simulink model "HalfCar"  (R2024b)
settings: Solver=VariableStepAuto  StartTime=0.0  StopTime=20  RelTol=1e-3
libraries: simulink x12
settings Model: Creator=Seb  LastModifiedBy=sebam

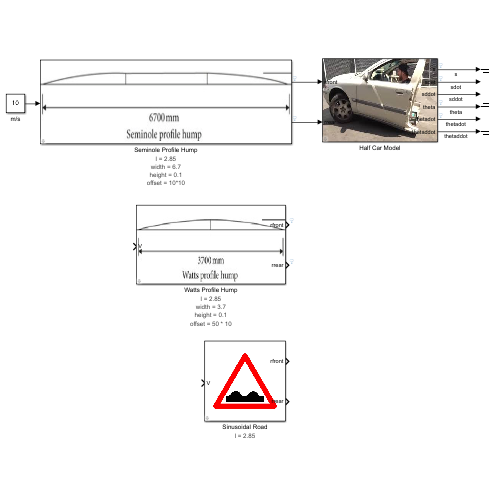
[thumbnail: Simulink's stored preview of the top-level diagram]
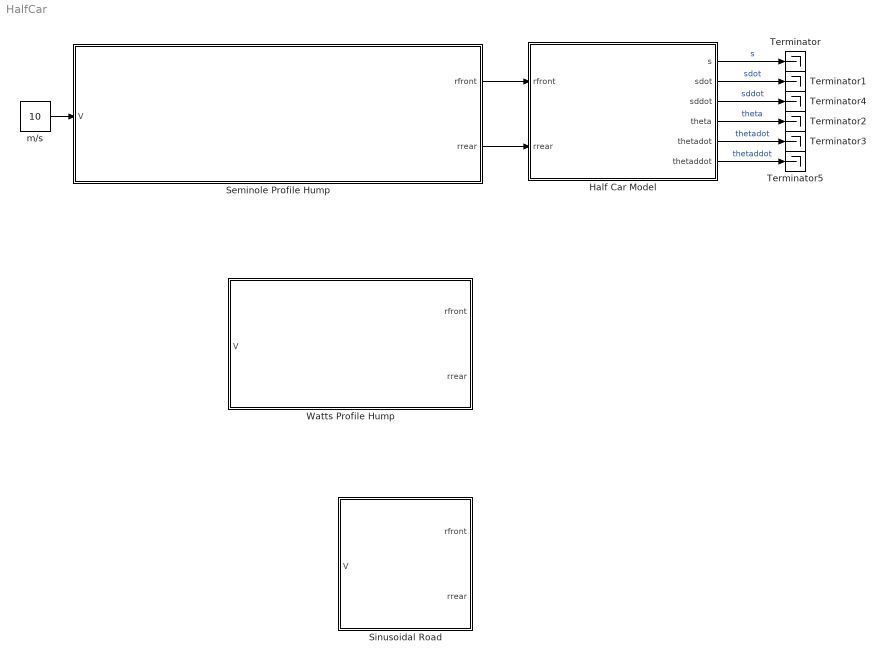
== system HalfCar ==
  Half Car Model : Subsystem
      mask Display: image('car.jpg');
  Seminole Profile Hump : Subsystem  mask{l=2.85, width=6.7, height=0.1, offset=10*10}
      mask prompts: l "Wheelbase (l)"; width "Hump Width (width)"; height "Hump Height (height)"; offset "Hump Offset (offset)"
      settings: AttributesFormatString=|
      | l = %<l>
      | width = %<width>
      | height = %<height>
      | offset = %<offset>
      mask Display: image('seminole.png');
  Sinusoidal Road : Subsystem  mask{l=2.85}
      mask prompts: l "Wheelbase (l)"
      settings: AttributesFormatString=l = %<l>
      mask Display: image('road.jpg');
  Terminator{,1..5} (6 alike) : Terminator
  Watts Profile Hump : Subsystem  mask{l=2.85, width=3.7, height=0.1, offset=50 * 10}
      mask prompts: l "Wheelbase (l)"; width "Hump Width (width)"; height "Hump Height (height)"; offset "Hump Offset (offset)"
      settings: AttributesFormatString=|
      | l = %<l>
      | width = %<width>
      | height = %<height>
      | offset = %<offset>
      mask Display: image('watt.png');
  m/s : Constant  Value=10
  wires:
  Half Car Model/1(s) -> Terminator/1  "s"
  Half Car Model/2(sdot) -> Terminator1/1  "sdot"
  Half Car Model/4(theta) -> Terminator2/1  "theta"
  Half Car Model/5(thetadot) -> Terminator3/1  "thetadot"
  m/s/1 -> Seminole Profile Hump/1(V)
  Seminole Profile Hump/1(rfront) -> Half Car Model/1(rfront)
  Seminole Profile Hump/2(rrear) -> Half Car Model/2(rrear)
  Half Car Model/3(sddot) -> Terminator4/1  "sddot"
  Half Car Model/6(thetaddot) -> Terminator5/1  "thetaddot"

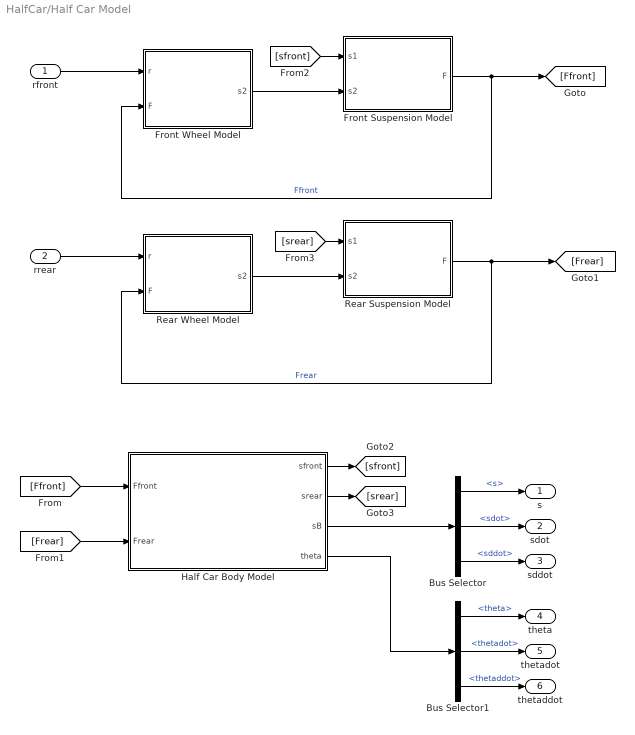
== system HalfCar/Half Car Model ==
  rfront : Inport
  rrear : Inport  Port=2
  Bus Selector : BusSelector  OutputSignals=s,sdot,sddot
  Bus Selector1 : BusSelector  OutputSignals=theta,thetadot,thetaddot
  Front Suspension Model : Subsystem  mask{ks=2e4, k2=20*2e4, x0=0.2, ce=1200, cc=600}
      mask prompts: ks "Spring Stiffness (ks)"; k2 "Spring Hardening Stiffness (k2)"; x0 "Spring Hardening Location (x0)"; ce "Damping Rate Extension (cse)"; cc "Damping Rate Compression (csc)"
      settings: AttributesFormatString=|
      | ks = %<ks>
      | k2 = %<k2>
      | x0 = %<x0>
      | ce = %<ce>
      | cc = %<cc>
      mask Display: fprintf("Suspension\nModel")
  Front Wheel Model : Subsystem  mask{m2=20, g=9.81, kT=14e4}
      mask prompts: m2 "Mass (m2)"; g "Gravity (g)"; kT "Wheel Stiffness (kT)"
      settings: AttributesFormatString=|
      | g = %<g>
      | kT = %<kT>
      | m2 = %<m2>
      mask Display: fprintf("Wheel\nModel")
  Half Car Body Model : Subsystem  mask{mB=700, IB=650, g=9.81, a=1.35, b=1.5}
      mask prompts: mB "Mass (mB)"; IB "Moment of Inertia (IB)"; g "Gravity (g)"; a "Length A (a)"; b "Length B (b)"
      settings: AttributesFormatString=|
      | mB = %<mB>
      | IB = %<IB>
      | g = %<g>
      | a = %<a>
      | b = %<b>
      mask Display: fprintf("Half Car\nBody Model")
  Rear Suspension Model : Subsystem  mask{ks=2e4, k2=20*2e4, x0=0.2, ce=1200, cc=600}
      mask prompts: ks "Spring Stiffness (ks)"; k2 "Spring Hardening Stiffness (k2)"; x0 "Spring Hardening Location (x0)"; ce "Damping Rate Extension (cse)"; cc "Damping Rate Compression (csc)"
      settings: AttributesFormatString=|
      | ks = %<ks>
      | k2 = %<k2>
      | x0 = %<x0>
      | ce = %<ce>
      | cc = %<cc>
      mask Display: fprintf("Suspension\nModel")
  Rear Wheel Model : Subsystem  mask{m2=20, g=9.81, kT=14e4}
      mask prompts: m2 "Mass (m2)"; g "Gravity (g)"; kT "Wheel Stiffness (kT)"
      settings: AttributesFormatString=|
      | g = %<g>
      | kT = %<kT>
      | m2 = %<m2>
      mask Display: fprintf("Wheel\nModel")
  s : Outport
  sdot : Outport  Port=2
  sddot : Outport  Port=3
  theta : Outport  Port=4
  thetadot : Outport  Port=5
  thetaddot : Outport  Port=6
  wires:
  Front Wheel Model/1(s2) -> Front Suspension Model/2(s2)
  Half Car Body Model/3(sB) -> Bus Selector/1
  Front Suspension Model/1(F) -> [Ffront], Front Wheel Model/2(F)  "Ffront"
  Bus Selector/2 -> sdot/1  "<sdot>"
  Half Car Body Model/4(theta) -> Bus Selector1/1
  Bus Selector1/1 -> theta/1  "<theta>"
  rfront/1 -> Front Wheel Model/1(r)
  Bus Selector1/2 -> thetadot/1  "<thetadot>"
  rrear/1 -> Rear Wheel Model/1(r)
  Bus Selector/1 -> s/1  "<s>"
  Rear Suspension Model/1(F) -> [Frear], Rear Wheel Model/2(F)  "Frear"
  Rear Wheel Model/1(s2) -> Rear Suspension Model/2(s2)
  [Ffront] -> Half Car Body Model/1(Ffront)
  [Frear] -> Half Car Body Model/2(Frear)
  Half Car Body Model/1(sfront) -> [sfront]
  Half Car Body Model/2(srear) -> [srear]
  [sfront] -> Front Suspension Model/1(s1)
  [srear] -> Rear Suspension Model/1(s1)
  Bus Selector/3 -> sddot/1  "<sddot>"
  Bus Selector1/3 -> thetaddot/1  "<thetaddot>"

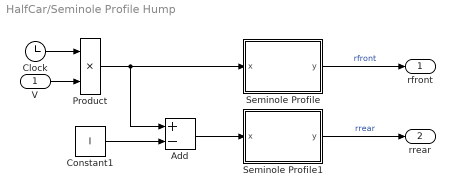
== system HalfCar/Seminole Profile Hump ==
  V : Inport
  Add : Sum  Inputs=+-
  Clock : Clock
  Constant1 : Constant  Value=l
  Product : Product
  Seminole Profile : Subsystem
  Seminole Profile1 : Subsystem
  rfront : Outport
  rrear : Outport  Port=2
  wires:
  V/1 -> Product/2
  Seminole Profile1/1(y) -> rrear/1  "rrear"
  Constant1/1 -> Add/2
  Product/1 -> Seminole Profile/1(x), Add/1
  Add/1 -> Seminole Profile1/1(x)
  Seminole Profile/1(y) -> rfront/1  "rfront"
  Clock/1 -> Product/1

== system HalfCar/Sinusoidal Road ==
  V : Inport
  Add : Sum  Inputs=+-
  Clock : Clock
  Constant1 : Constant  Value=l
  Product : Product
  Sine Wave Function : Sin  TimeSource=Use external signal  Amplitude=0.01  Frequency=2*pi  SampleTime=0
      settings: AttributesFormatString=|
      | Amplitude = %<Amplitude>
      | Frequency = %<Frequency>
  Sine Wave Function1 : Sin  TimeSource=Use external signal  Amplitude=0.01  Frequency=2*pi  SampleTime=0
      settings: AttributesFormatString=|
      | Amplitude = %<Amplitude>
      | Frequency = %<Frequency>
  rfront : Outport
  rrear : Outport  Port=2
  wires:
  Sine Wave Function1/1 -> rrear/1  "rrear"
  V/1 -> Product/2
  Sine Wave Function/1 -> rfront/1  "rfront"
  Add/1 -> Sine Wave Function1/1
  Constant1/1 -> Add/2
  Product/1 -> Add/1, Sine Wave Function/1
  Clock/1 -> Product/1

== system HalfCar/Watts Profile Hump ==
  V : Inport
  Add : Sum  Inputs=+-
  Clock : Clock
  Constant1 : Constant  Value=l
  Product : Product
  Watts Profile : Subsystem
  Watts Profile1 : Subsystem
  rfront : Outport
  rrear : Outport  Port=2
  wires:
  Clock/1 -> Product/1
  Watts Profile/1(y) -> rfront/1  "rfront"
  Add/1 -> Watts Profile1/1(x)
  Product/1 -> Watts Profile/1(x), Add/1
  Constant1/1 -> Add/2
  Watts Profile1/1(y) -> rrear/1  "rrear"
  V/1 -> Product/2

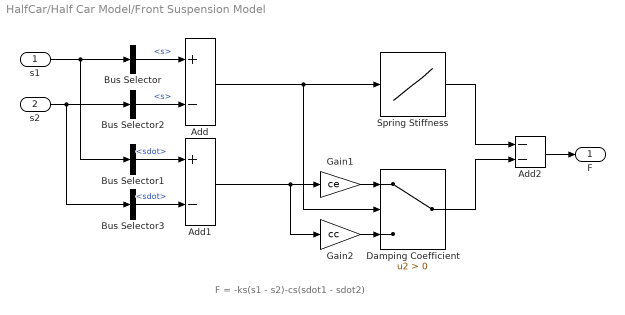
== system HalfCar/Half Car Model/Front Suspension Model ==
  note: F = -ks(s1 - s2)-cs(sdot1 - sdot2)
  s1 : Inport
  s2 : Inport  Port=2
  Add : Sum  Inputs=+-
  Add1 : Sum  Inputs=+-
  Add2 : Sum  Inputs=--
  Bus Selector : BusSelector  OutputSignals=s
  Bus Selector1 : BusSelector  OutputSignals=sdot
  Bus Selector2 : BusSelector  OutputSignals=s
  Bus Selector3 : BusSelector  OutputSignals=sdot
  Damping Coefficient : Switch  Criteria=u2 > Threshold  SaturateOnIntegerOverflow=off  InputSameDT=off
  Gain1 : Gain  Gain=ce
  Gain2 : Gain  Gain=cc
  Spring Stiffness : Lookup_n-D  NumberOfTableDimensions=1  BreakpointsForDimension1=[-2*x0, -x0, x0, 2*x0]  Table=[-(ks+k2)*x0, -ks*x0, ks*x0, (ks+k2)*x0]  InternalRulePriority=Speed  RndMeth=Simplest
  F : Outport
  wires:
  s1/1 -> Bus Selector1/1, Bus Selector/1
  s2/1 -> Bus Selector2/1, Bus Selector3/1
  Add/1 -> Spring Stiffness/1, Damping Coefficient/2
  Bus Selector/1 -> Add/1  "<s>"
  Bus Selector1/1 -> Add1/1  "<sdot>"
  Add1/1 -> Gain2/1, Gain1/1
  Spring Stiffness/1 -> Add2/1
  Damping Coefficient/1 -> Add2/2
  Add2/1 -> F/1
  Bus Selector2/1 -> Add/2  "<s>"
  Bus Selector3/1 -> Add1/2  "<sdot>"
  Gain1/1 -> Damping Coefficient/1
  Gain2/1 -> Damping Coefficient/3

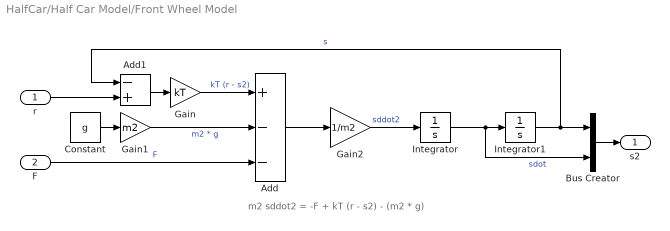
== system HalfCar/Half Car Model/Front Wheel Model ==
  note: m2 sddot2 = -F + kT (r - s2) - (m2 * g)
  r : Inport
  F : Inport  Port=2
  Add : Sum  Inputs=+--
  Add1 : Sum  Inputs=-+
  Bus Creator : BusCreator  Inputs=2
  Constant : Constant  Value=g
  Gain : Gain  Gain=kT
  Gain1 : Gain  Gain=m2
  Gain2 : Gain  Gain=1/m2
  Integrator : Integrator
  Integrator1 : Integrator
  s2 : Outport
  wires:
  r/1 -> Add1/2
  Bus Creator/1 -> s2/1
  Gain2/1 -> Integrator/1  "sddot2"
  Constant/1 -> Gain1/1
  Integrator/1 -> Bus Creator/2, Integrator1/1  "sdot"
  Add/1 -> Gain2/1
  Integrator1/1 -> Add1/1, Bus Creator/1  "s"
  Gain1/1 -> Add/2  "m2 * g"
  F/1 -> Add/3  "F"
  Gain/1 -> Add/1  "kT (r - s2)"
  Add1/1 -> Gain/1

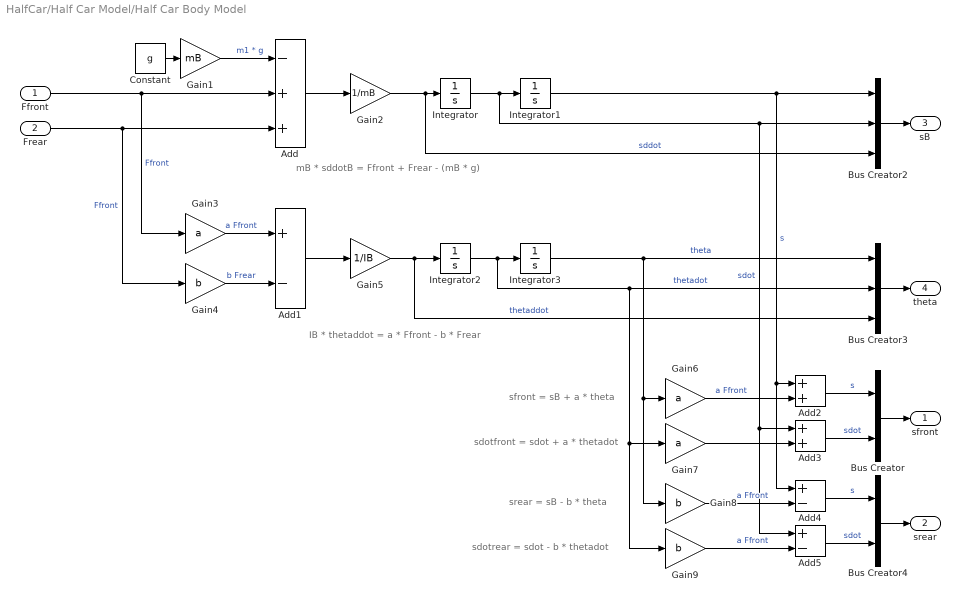
== system HalfCar/Half Car Model/Half Car Body Model ==
  note: sfront = sB + a * theta
  note: IB * thetaddot = a * Ffront - b * Frear
  note: mB * sddotB = Ffront + Frear - (mB * g)
  note: sdotfront = sdot + a * thetadot
  note: srear = sB - b * theta
  note: sdotrear = sdot - b * thetadot
  Ffront : Inport
  Frear : Inport  Port=2
  Add : Sum  Inputs=-++
  Add1 : Sum  Inputs=+-
  Add2 : Sum
  Add3 : Sum
  Add4 : Sum  Inputs=+-
  Add5 : Sum  Inputs=+-
  Bus Creator : BusCreator  Inputs=2
  Bus Creator2 : BusCreator  Inputs=3
  Bus Creator3 : BusCreator  Inputs=3
  Bus Creator4 : BusCreator  Inputs=2
  Constant : Constant  Value=g
  Gain1 : Gain  Gain=mB
  Gain2 : Gain  Gain=1/mB
  Gain3 : Gain  Gain=a
  Gain4 : Gain  Gain=b
  Gain5 : Gain  Gain=1/IB
  Gain6 : Gain  Gain=a
  Gain7 : Gain  Gain=a
  Gain8 : Gain  Gain=b
  Gain9 : Gain  Gain=b
  Integrator{,1..3} (4 alike) : Integrator
  sfront : Outport
  srear : Outport  Port=2
  sB : Outport  Port=3
  theta : Outport  Port=4
  wires:
  Integrator1/1 -> Add4/1, Add2/1, Bus Creator2/1  "s"
  Add/1 -> Gain2/1
  Constant/1 -> Gain1/1
  Gain1/1 -> Add/1  "m1 * g"
  Gain2/1 -> Bus Creator2/3, Integrator/1  "sddot"
  Bus Creator/1 -> sfront/1
  Bus Creator4/1 -> srear/1
  Bus Creator2/1 -> sB/1
  Integrator/1 -> Integrator1/1, Add5/1, Add3/1, Bus Creator2/2  "sdot"
  Add3/1 -> Bus Creator/2  "sdot"
  Gain3/1 -> Add1/1  "a Ffront"
  Gain4/1 -> Add1/2  "b Frear"
  Add1/1 -> Gain5/1
  Gain5/1 -> Bus Creator3/3, Integrator2/1  "thetaddot"
  Integrator2/1 -> Gain9/1, Gain7/1, Bus Creator3/2, Integrator3/1  "thetadot"
  Integrator3/1 -> Gain8/1, Gain6/1, Bus Creator3/1  "theta"
  Bus Creator3/1 -> theta/1
  Add2/1 -> Bus Creator/1  "s"
  Gain6/1 -> Add2/2  "a Ffront"
  Gain7/1 -> Add3/2
  Add4/1 -> Bus Creator4/1  "s"
  Add5/1 -> Bus Creator4/2  "sdot"
  Gain8/1 -> Add4/2  "a Ffront"
  Gain9/1 -> Add5/2  "a Ffront"
  Ffront/1 -> Gain3/1, Add/2  "Ffront"
  Frear/1 -> Gain4/1, Add/3  "Ffront"

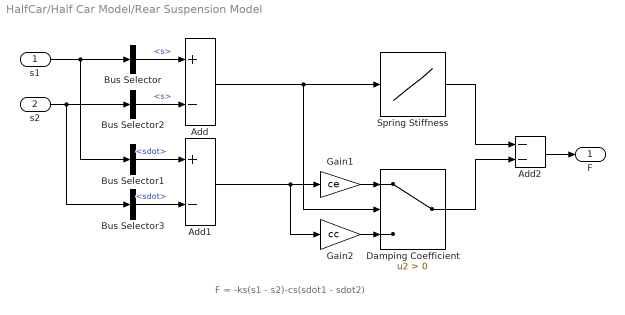
== system HalfCar/Half Car Model/Rear Suspension Model ==
  note: F = -ks(s1 - s2)-cs(sdot1 - sdot2)
  s1 : Inport
  s2 : Inport  Port=2
  Add : Sum  Inputs=+-
  Add1 : Sum  Inputs=+-
  Add2 : Sum  Inputs=--
  Bus Selector : BusSelector  OutputSignals=s
  Bus Selector1 : BusSelector  OutputSignals=sdot
  Bus Selector2 : BusSelector  OutputSignals=s
  Bus Selector3 : BusSelector  OutputSignals=sdot
  Damping Coefficient : Switch  Criteria=u2 > Threshold  SaturateOnIntegerOverflow=off  InputSameDT=off
  Gain1 : Gain  Gain=ce
  Gain2 : Gain  Gain=cc
  Spring Stiffness : Lookup_n-D  NumberOfTableDimensions=1  BreakpointsForDimension1=[-2*x0, -x0, x0, 2*x0]  Table=[-(ks+k2)*x0, -ks*x0, ks*x0, (ks+k2)*x0]  InternalRulePriority=Speed  RndMeth=Simplest
  F : Outport
  wires:
  Damping Coefficient/1 -> Add2/2
  Add1/1 -> Gain2/1, Gain1/1
  Add2/1 -> F/1
  Bus Selector/1 -> Add/1  "<s>"
  Bus Selector2/1 -> Add/2  "<s>"
  Bus Selector1/1 -> Add1/1  "<sdot>"
  Bus Selector3/1 -> Add1/2  "<sdot>"
  s2/1 -> Bus Selector2/1, Bus Selector3/1
  Gain2/1 -> Damping Coefficient/3
  s1/1 -> Bus Selector1/1, Bus Selector/1
  Gain1/1 -> Damping Coefficient/1
  Add/1 -> Spring Stiffness/1, Damping Coefficient/2
  Spring Stiffness/1 -> Add2/1

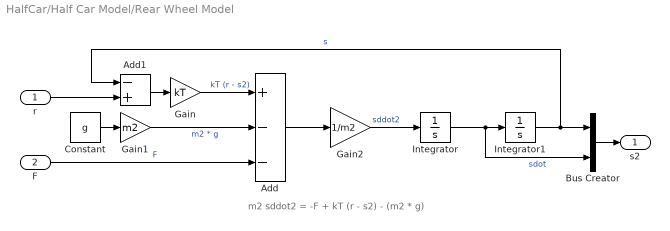
== system HalfCar/Half Car Model/Rear Wheel Model ==
  note: m2 sddot2 = -F + kT (r - s2) - (m2 * g)
  r : Inport
  F : Inport  Port=2
  Add : Sum  Inputs=+--
  Add1 : Sum  Inputs=-+
  Bus Creator : BusCreator  Inputs=2
  Constant : Constant  Value=g
  Gain : Gain  Gain=kT
  Gain1 : Gain  Gain=m2
  Gain2 : Gain  Gain=1/m2
  Integrator : Integrator
  Integrator1 : Integrator
  s2 : Outport
  wires:
  Add1/1 -> Gain/1
  Gain/1 -> Add/1  "kT (r - s2)"
  F/1 -> Add/3  "F"
  Gain1/1 -> Add/2  "m2 * g"
  Integrator1/1 -> Bus Creator/1, Add1/1  "s"
  Add/1 -> Gain2/1
  Integrator/1 -> Integrator1/1, Bus Creator/2  "sdot"
  Constant/1 -> Gain1/1
  Gain2/1 -> Integrator/1  "sddot2"
  Bus Creator/1 -> s2/1
  r/1 -> Add1/2

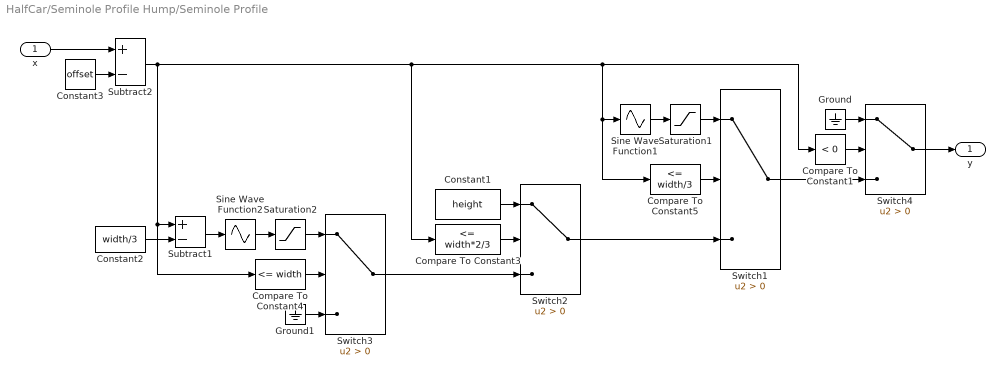
== system HalfCar/Seminole Profile Hump/Seminole Profile ==
  x : Inport
  Compare To Constant1 : simulink/Logic and Bit Operations/Compare To Constant  relop=<  const=0  OutDataTypeStr=boolean
  Compare To Constant3 : simulink/Logic and Bit Operations/Compare To Constant  relop=<=  const=width*2/3  OutDataTypeStr=boolean
  Compare To Constant4 : simulink/Logic and Bit Operations/Compare To Constant  relop=<=  const=width  OutDataTypeStr=boolean
  Compare To Constant5 : simulink/Logic and Bit Operations/Compare To Constant  relop=<=  const=width/3  OutDataTypeStr=boolean
  Constant1 : Constant  Value=height
  Constant2 : Constant  Value=width/3
  Constant3 : Constant  Value=offset
  Ground : Ground
  Ground1 : Ground
  Saturation1 : Saturate  UpperLimit=height  LowerLimit=0
  Saturation2 : Saturate  UpperLimit=height  LowerLimit=0
  Sine Wave Function1 : Sin  TimeSource=Use external signal  Amplitude=height  Frequency=(2*pi)/(width*4/3)  SampleTime=0
  Sine Wave Function2 : Sin  TimeSource=Use external signal  Amplitude=height  Frequency=(2*pi)/(width*4/3)  SampleTime=0
  Subtract1 : Sum  Inputs=+-
  Subtract2 : Sum  Inputs=+-
  Switch{1..4} (4 alike) : Switch  Criteria=u2 > Threshold  SaturateOnIntegerOverflow=off  InputSameDT=off
  y : Outport
  wires:
  Constant2/1 -> Subtract1/2
  Saturation2/1 -> Switch3/1
  Ground1/1 -> Switch3/3
  Constant1/1 -> Switch2/1
  Compare To Constant3/1 -> Switch2/2
  Compare To Constant4/1 -> Switch3/2
  Switch3/1 -> Switch2/3
  Switch2/1 -> Switch1/3
  Sine Wave Function2/1 -> Saturation2/1
  Subtract2/1 -> Compare To Constant3/1, Compare To Constant5/1, Sine Wave Function1/1, Compare To Constant1/1, Compare To Constant4/1, Subtract1/1
  Saturation1/1 -> Switch1/1
  Sine Wave Function1/1 -> Saturation1/1
  Subtract1/1 -> Sine Wave Function2/1
  Compare To Constant5/1 -> Switch1/2
  x/1 -> Subtract2/1
  Constant3/1 -> Subtract2/2
  Switch1/1 -> Switch4/3
  Switch4/1 -> y/1
  Compare To Constant1/1 -> Switch4/2
  Ground/1 -> Switch4/1

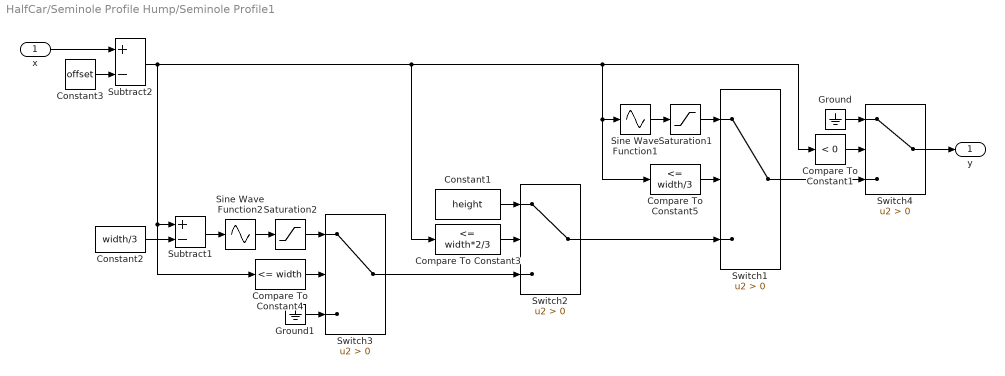
== system HalfCar/Seminole Profile Hump/Seminole Profile1 ==
  x : Inport
  Compare To Constant1 : simulink/Logic and Bit Operations/Compare To Constant  relop=<  const=0  OutDataTypeStr=boolean
  Compare To Constant3 : simulink/Logic and Bit Operations/Compare To Constant  relop=<=  const=width*2/3  OutDataTypeStr=boolean
  Compare To Constant4 : simulink/Logic and Bit Operations/Compare To Constant  relop=<=  const=width  OutDataTypeStr=boolean
  Compare To Constant5 : simulink/Logic and Bit Operations/Compare To Constant  relop=<=  const=width/3  OutDataTypeStr=boolean
  Constant1 : Constant  Value=height
  Constant2 : Constant  Value=width/3
  Constant3 : Constant  Value=offset
  Ground : Ground
  Ground1 : Ground
  Saturation1 : Saturate  UpperLimit=height  LowerLimit=0
  Saturation2 : Saturate  UpperLimit=height  LowerLimit=0
  Sine Wave Function1 : Sin  TimeSource=Use external signal  Amplitude=height  Frequency=(2*pi)/(width*4/3)  SampleTime=0
  Sine Wave Function2 : Sin  TimeSource=Use external signal  Amplitude=height  Frequency=(2*pi)/(width*4/3)  SampleTime=0
  Subtract1 : Sum  Inputs=+-
  Subtract2 : Sum  Inputs=+-
  Switch{1..4} (4 alike) : Switch  Criteria=u2 > Threshold  SaturateOnIntegerOverflow=off  InputSameDT=off
  y : Outport
  wires:
  Constant2/1 -> Subtract1/2
  Saturation2/1 -> Switch3/1
  Ground1/1 -> Switch3/3
  Constant1/1 -> Switch2/1
  Compare To Constant3/1 -> Switch2/2
  Compare To Constant4/1 -> Switch3/2
  Switch3/1 -> Switch2/3
  Switch2/1 -> Switch1/3
  Sine Wave Function2/1 -> Saturation2/1
  Subtract2/1 -> Compare To Constant3/1, Compare To Constant5/1, Sine Wave Function1/1, Compare To Constant1/1, Compare To Constant4/1, Subtract1/1
  Saturation1/1 -> Switch1/1
  Sine Wave Function1/1 -> Saturation1/1
  Subtract1/1 -> Sine Wave Function2/1
  Compare To Constant5/1 -> Switch1/2
  x/1 -> Subtract2/1
  Constant3/1 -> Subtract2/2
  Switch1/1 -> Switch4/3
  Switch4/1 -> y/1
  Compare To Constant1/1 -> Switch4/2
  Ground/1 -> Switch4/1

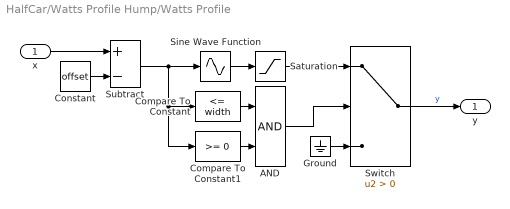
== system HalfCar/Watts Profile Hump/Watts Profile ==
  x : Inport
  AND : Logic  AllPortsSameDT=off  OutDataTypeStr=boolean
  Compare To Constant : simulink/Logic and Bit Operations/Compare To Constant  relop=<=  const=width  OutDataTypeStr=boolean
  Compare To Constant1 : simulink/Logic and Bit Operations/Compare To Constant  relop=>=  const=0  OutDataTypeStr=boolean
  Constant : Constant  Value=offset
  Ground : Ground
  Saturation : Saturate  UpperLimit=height  LowerLimit=0
  Sine Wave Function : Sin  TimeSource=Use external signal  Amplitude=height  Frequency=(2*pi)/(width*2)  SampleTime=0
  Subtract : Sum  Inputs=+-
  Switch : Switch  Criteria=u2 > Threshold  SaturateOnIntegerOverflow=off  InputSameDT=off
  y : Outport
  wires:
  Saturation/1 -> Switch/1
  Compare To Constant/1 -> AND/1
  Sine Wave Function/1 -> Saturation/1
  Ground/1 -> Switch/3
  Subtract/1 -> Compare To Constant1/1, Compare To Constant/1, Sine Wave Function/1
  Switch/1 -> y/1  "y"
  x/1 -> Subtract/1
  Compare To Constant1/1 -> AND/2
  AND/1 -> Switch/2
  Constant/1 -> Subtract/2

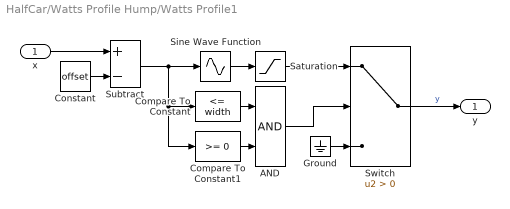
== system HalfCar/Watts Profile Hump/Watts Profile1 ==
  x : Inport
  AND : Logic  AllPortsSameDT=off  OutDataTypeStr=boolean
  Compare To Constant : simulink/Logic and Bit Operations/Compare To Constant  relop=<=  const=width  OutDataTypeStr=boolean
  Compare To Constant1 : simulink/Logic and Bit Operations/Compare To Constant  relop=>=  const=0  OutDataTypeStr=boolean
  Constant : Constant  Value=offset
  Ground : Ground
  Saturation : Saturate  UpperLimit=height  LowerLimit=0
  Sine Wave Function : Sin  TimeSource=Use external signal  Amplitude=height  Frequency=(2*pi)/(width*2)  SampleTime=0
  Subtract : Sum  Inputs=+-
  Switch : Switch  Criteria=u2 > Threshold  SaturateOnIntegerOverflow=off  InputSameDT=off
  y : Outport
  wires:
  Constant/1 -> Subtract/2
  AND/1 -> Switch/2
  Compare To Constant1/1 -> AND/2
  x/1 -> Subtract/1
  Switch/1 -> y/1  "y"
  Subtract/1 -> Sine Wave Function/1, Compare To Constant/1, Compare To Constant1/1
  Ground/1 -> Switch/3
  Sine Wave Function/1 -> Saturation/1
  Compare To Constant/1 -> AND/1
  Saturation/1 -> Switch/1
